simulink model "qam_1"  (Simulink 5.1)
settings: Solver=ode45  StartTime=0.0  StopTime=2  RelTol=1e-3
values from neighbouring files (symbols this model uses):
  fc = 0.2    [TP_fdesign1.m]    (also in TP_fdesign2.m; band4.m = 2000)
  h0 = zeros(1,L)    [G722_1.m]    (also in audio_test1.m = han(:,1); audio_test2.m = han(:,1); band4.m = fir1(nf, 2*ftp))
  htp = fir1(64, 0.6)    [adaptiv_3.m]
  nf = 256    [band4.m]    (also in block_lms_.m = 16)
  Ts = 1/fs    (= 6.25e-05)    [G722_1.m]    (also in adaptiv_2.m = 0.001; adaptiv_3.m = 0.001; adaptiv_4.m = 0.001; adaptiv_5.m = 0.001)
undefined symbols (not defined in the file or in its folder): get
libraries: dspsigops x6, dspsrcs4 x1, dspsnks4 x1
settings Model: Creator=svenhoffmann  LastModifiedBy=svenhoffmann  ExtModeAutoUpdateStatusClock=off  BooleanDataType=on  ProdHWDeviceType=Microprocessor

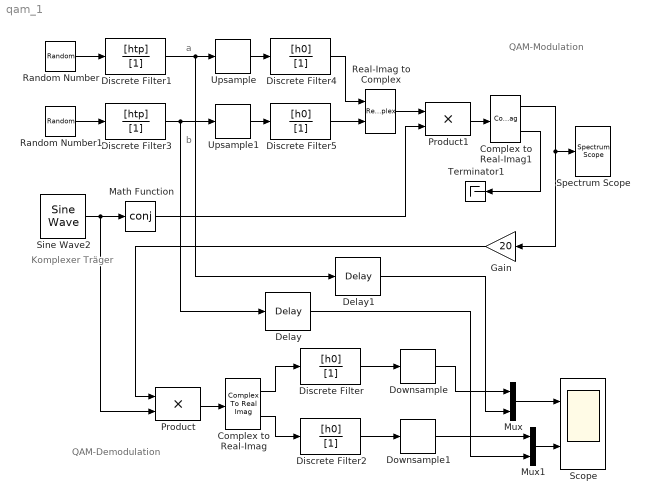
== system qam_1 ==
  note: QAM-Modulation
  note: QAM-Demodulation
  note: Komplexer
      | Träger
  note: a
  note: b
  Complex to Real-Imag : ComplexToRealImag
  Complex to Real-Imag1 : ComplexToRealImag
  Delay : dspsigops/Delay  dly_unit=Samples  delay=fix(nf/20)+10  ic_detail=off  dif_ic_for_ch=off  dif_ic_for_dly=off  ic=0  reset_popup=None
  Delay1 : dspsigops/Delay  dly_unit=Samples  delay=fix(nf/20)+10  ic_detail=off  dif_ic_for_ch=off  dif_ic_for_dly=off  ic=0  reset_popup=None
  Discrete Filter{,2,4..5} (4 alike) : DiscreteFilter  Numerator=[h0]  Denominator=[1]  SampleTime=Ts
  Discrete Filter1 : DiscreteFilter  Numerator=[htp]  Denominator=[1]  SampleTime=Ts*10
  Discrete Filter3 : DiscreteFilter  Numerator=[htp]  Denominator=[1]  SampleTime=Ts*10
  Downsample : dspsigops/Downsample  N=10  phase=0  ic=0  smode=Allow multirate  fmode=Maintain input frame size
  Downsample1 : dspsigops/Downsample  N=10  phase=0  ic=0  smode=Allow multirate  fmode=Maintain input frame size
  Gain : Gain  Orientation=left  Gain=20  SaturateOnIntegerOverflow=on
  Math Function : Math  Operator=conj
  Mux : Mux  Inputs=2
  Mux1 : Mux  Inputs=2
  Product : Product  SaturateOnIntegerOverflow=on
  Product1 : Product  SaturateOnIntegerOverflow=on
  Random Number : RandomNumber  SampleTime=0
  Random Number1 : RandomNumber  Seed=18752  SampleTime=0
  Real-Imag to Complex : RealImagToComplex
  Scope : Scope  NumInputPorts=2
      settings: YMin=-1.2~-1.2  YMax=1.2~1.2
  Sine Wave2 : dspsrcs4/Sine Wave  Amplitude=1  Frequency=fc  Phase=0  SampleMode=Discrete  OutComplex=Complex  CompMethod=Trigonometric fcn  TableSize=Speed  SampleTime=Ts  SamplesPerFrame=1  dataType=double  wordLen=16  udDataType=sfix(16)  fracBitsMode=Best precision  numFracBits=15  ResetState=Restart at time zero
      settings: additionalParams=on
  Spectrum Scope : dspsnks4/Spectrum Scope  ScopeProperties=on  Domain=Frequency  HorizSpan=1  UseBuffer=on  BufferSize=256  Overlap=64  inpFftLenInherit=off  FFTlength=128  numAvg=10  DisplayProperties=off  AxisGrid=on  Memory=off  FrameNumber=on  AxisLegend=off  AxisZoom=off  OpenScopeAtSimStart=on  OpenScopeImmediately=off  FigPos=get(0,'defaultfigureposition')  AxisProperties=off  XUnits=Hertz  XRange=[0...Fs]  InheritXIncr=off  XIncr=Ts  XLabel=Samples  YUnits=dB  YLabel=Magnitude, dB  LineProperties=off
      settings: YMin=-141.470991898451  YMax=-14.4727896416515
  Terminator1 : Terminator
  Upsample : dspsigops/Upsample  N=10  phase=0  ic=0  mode=Maintain input frame size
  Upsample1 : dspsigops/Upsample  N=10  phase=0  ic=0  mode=Maintain input frame size
  wires:
  Product/1 -> Complex to Real-Imag/1
  Complex to Real-Imag/1 -> Discrete Filter/1
  Complex to Real-Imag/2 -> Discrete Filter2/1
  Discrete Filter/1 -> Downsample/1
  Mux/1 -> Scope/1
  Sine Wave2/1 -> Product/2, Math Function/1
  Product1/1 -> Complex to Real-Imag1/1
  Discrete Filter1/1 -> Upsample/1, Delay1/1
  Discrete Filter3/1 -> Delay/1, Upsample1/1
  Real-Imag to Complex/1 -> Product1/1
  Mux1/1 -> Scope/2
  Discrete Filter2/1 -> Downsample1/1
  Delay/1 -> Mux1/2
  Delay1/1 -> Mux/2
  Downsample/1 -> Mux/1
  Downsample1/1 -> Mux1/1
  Math Function/1 -> Product1/2
  Complex to Real-Imag1/1 -> Spectrum Scope/1, Gain/1
  Complex to Real-Imag1/2 -> Terminator1/1
  Random Number/1 -> Discrete Filter1/1
  Random Number1/1 -> Discrete Filter3/1
  Gain/1 -> Product/1
  Upsample/1 -> Discrete Filter4/1
  Discrete Filter4/1 -> Real-Imag to Complex/1
  Upsample1/1 -> Discrete Filter5/1
  Discrete Filter5/1 -> Real-Imag to Complex/2
